simulink model "vehicle_par"  (R2017a)
settings: Solver=FixedStepDiscrete  StartTime=0.0  StopTime=inf  FixedStep=abs(Ts)  RelTol=1e-3
InitFcn:
  | if ~exist('Ts')
  |     Ts = 1;
  | end
undefined symbols (not defined in the file or in its folder): elvio_cycle_wltp_3b
libraries: elvio x15
settings Model: Creator=tstef  LastModifiedBy=elts2

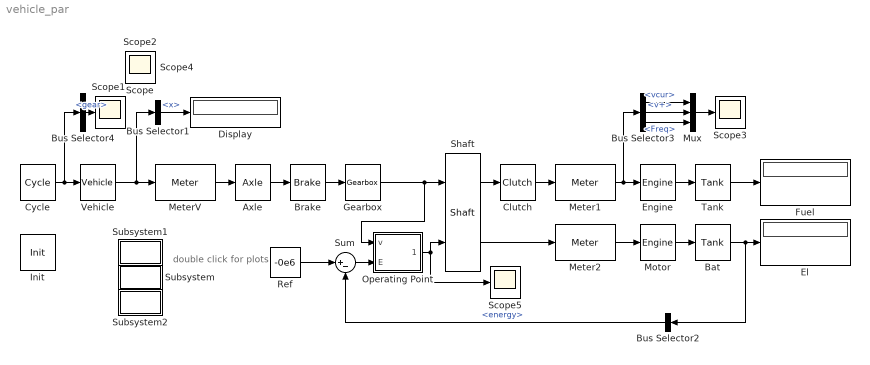
== system vehicle_par ==
  note: double click
      | for plots
  Axle : elvio/Drive/Axle  radius=0.3  ratio=4  factor=0.1  FromTag1=Axle1  GotoTag1=MeterV1
  Bat : elvio/Drive/Tank  GotoTag1=Motor1
  Brake : elvio/Drive/Brake  Tbrake=5000  FromTag1=Brake1  GotoTag1=Axle1
  Bus Selector1 : BusSelector  OutputSignals=info.x
  Bus Selector2 : BusSelector  OutputSignals=energy
  Bus Selector3 : BusSelector  OutputSignals=vcur,v+,Freq
  Bus Selector4 : BusSelector  OutputSignals=gear
  Clutch : elvio/Drive/Clutch  speed=70  FromTag1=Clutch1  GotoTag1=Shaft1
  Cycle : elvio/Drive/Cycle  data=elvio_cycle_wltp_3b()
  Display : Display
  El : Display
  Engine : elvio/Drive/Engine  Tmax=110  Tmin=0  Tfrict=12  Ploss=1000  lossf=1.1  lossnorm=500e3  lossR=0.2  FromTag1=Engine1  GotoTag1=Meter11
  Fuel : Display
  Gearbox : elvio/Drive/Gearbox  gears=[4 2.5 1.8 1.2 0.9 0.9]  factor=0.1  FromTag1=Gearbox1  GotoTag1=Brake1
  Init : elvio/Drive/Init  Ts0=1
  Meter1 : elvio/Drive/Meter  FromTag1=Meter11  GotoTag1=Clutch1
  Meter2 : elvio/Drive/Meter  FromTag1=Meter21  GotoTag1=Shaft2
  MeterV : elvio/Drive/Meter  FromTag1=MeterV1  GotoTag1=Vehicle1
  Motor : elvio/Drive/Engine  Tmax=60  Tmin=-60  Tfrict=0.2  Ploss=100  lossf=0.01  lossnorm=2e6  lossR=0.05  FromTag1=Motor1  GotoTag1=Meter21
  Mux : Mux  Inputs=3
  Operating Point : Subsystem  mask(Operating Point){split=0.8, bias=20, kp=1e-4, Tmin=10, Tmax=100}
      mask prompts: split "Torque split [0-1]:"; bias "Torque bias [Nm];"; kp "Battery controller gain:"; Tmin "Min engine torque [Nm]:"; Tmax "Max engine torque [Nm]:"
      mask help: This block sets the torque operating point for the engine of a parallel hybrid.
  Ref : Constant  Value=-0e6
  Scope{,1..5} (6 alike) : Scope
      Scope4 mask Display: disp('1.484e+07')
  Shaft : elvio/Drive/Shaft  FromTag1=Shaft1  FromTag2=Shaft2  GotoTag1=Gearbox1
  Subsystem : Subsystem
      settings: OpenFcn=elvio_plot_scatter(logsout);
      mask Display: disp('Scatter')
  Subsystem1 : Subsystem
      settings: OpenFcn=elvio_plot_energy(logsout);
      mask Display: disp('Energy')
  Subsystem2 : Subsystem
      settings: OpenFcn=elvio_plot_sources(logsout);
      mask Display: disp('Sources')
  Sum : Sum  Inputs=|+-
  Tank : elvio/Drive/Tank  GotoTag1=Engine1
  Vehicle : elvio/Drive/Vehicle  m=1200  Froll=150  Aeff=[0.3:0.025:0.4]  n=[1 5]  FromTag1=Vehicle1
  wires:
  Vehicle/1 -> MeterV/1, Bus Selector1/1
  Engine/1 -> Tank/1
  Tank/1 -> Fuel/1
  Operating Point/1(Torque) -> Shaft/2, Scope5/1
  Motor/1 -> Bat/1
  Shaft/1 -> Clutch/1
  Bat/1 -> Bus Selector2/1, El/1
  Bus Selector1/1 -> Display/1  "<x>"
  Shaft/2 -> Meter2/1
  Meter2/1 -> Motor/1
  MeterV/1 -> Axle/1
  Bus Selector3/3 -> Mux/3  "<Freq>"
  Bus Selector3/2 -> Mux/2  "<v+>"
  Mux/1 -> Scope3/1
  Meter1/1 -> Bus Selector3/1, Engine/1
  Bus Selector3/1 -> Mux/1  "<vcur>"
  Cycle/1 -> Bus Selector4/1, Vehicle/1
  Bus Selector4/1 -> Scope1/1  "<gear>"
  Axle/1 -> Brake/1
  Brake/1 -> Gearbox/1
  Gearbox/1 -> Operating Point/1(v), Shaft/1
  Clutch/1 -> Meter1/1
  Sum/1 -> Operating Point/2(E)
  Ref/1 -> Sum/1
  Bus Selector2/1 -> Sum/2  "<energy>"

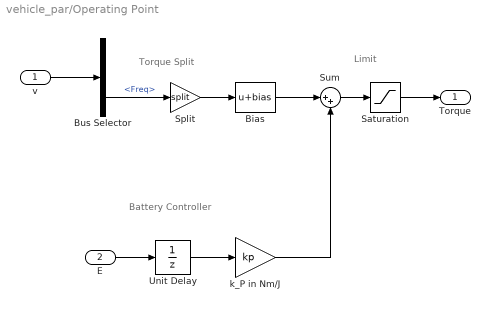
== system vehicle_par/Operating Point ==
  note: Limit
  note: Torque Split
  note: Battery Controller
  v : Inport
  E : Inport  Port=2
  Bias : Bias  Bias=bias
  Bus Selector : BusSelector  OutputSignals=vcur,Freq
  Saturation : Saturate  UpperLimit=Tmax  LowerLimit=Tmin
  Split : Gain  Gain=split
  Sum : Sum  Inputs=|++
  Unit Delay : UnitDelay  SampleTime=abs(Ts)
  k_P in Nm/J : Gain  Gain=kp
  Torque : Outport
  wires:
  Unit Delay/1 -> k_P in Nm/J/1
  E/1 -> Unit Delay/1
  k_P in Nm/J/1 -> Sum/2
  Saturation/1 -> Torque/1
  v/1 -> Bus Selector/1
  Bus Selector/2 -> Split/1  "<Freq>"
  Sum/1 -> Saturation/1
  Bias/1 -> Sum/1
  Split/1 -> Bias/1

== system vehicle_par/Subsystem ==

== system vehicle_par/Subsystem1 ==

== system vehicle_par/Subsystem2 ==
